simulink model "task_2"  (R2021b)
settings: Solver=daessc  StartTime=0.0  StopTime=3  FixedStep=1e-7  RelTol=1e-3
values from neighbouring files (symbols this model uses):
  x10 = 0    [env_practice_3.m]
  x20 = 10    [env_practice_3.m]
undefined symbols (not defined in the file or in its folder): magnitude
settings Model: Creator=79159  LastModifiedBy=79159
settings SolverCC: DaesscMode=Robust  ODENIntegrationMethod=ode1

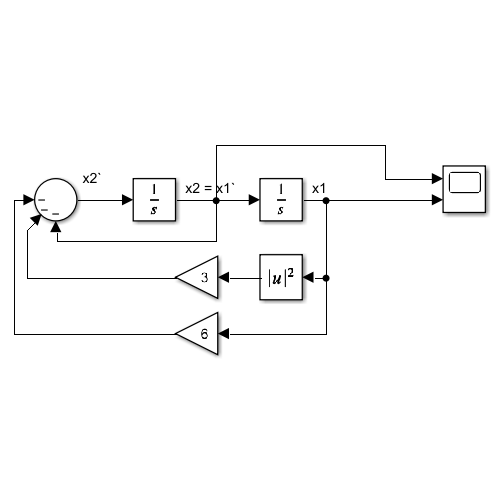
[thumbnail: Simulink's stored preview of the top-level diagram]
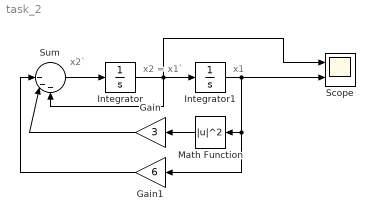
== system task_2 ==
  note: x2`
  note: x2 = x1`
  note: x1
  Gain : Gain  Gain=3
  Gain1 : Gain  Gain=6
  Integrator : Integrator  InitialCondition=x20
  Integrator1 : Integrator  InitialCondition=x10
  Math Function : Math  Operator=magnitude^2  SaturateOnIntegerOverflow=on
  Scope : Scope  NumInputPorts=2
  Sum : Sum  Inputs=||---
  wires:
  Sum/1 -> Integrator/1
  Integrator/1 -> Scope/1, Integrator1/1, Sum/3
  Integrator1/1 -> Gain1/1, Math Function/1, Scope/2
  Gain/1 -> Sum/2
  Math Function/1 -> Gain/1
  Gain1/1 -> Sum/1
